simulink library "DLR_BSW_lib"  (Simulink 8.1)
settings: Solver=ode45  SolverMode=SingleTasking  StartTime=0.0  StopTime=10.0  RelTol=1e-3
settings Model: Creator=Nathan  LastModifiedBy=Nathan

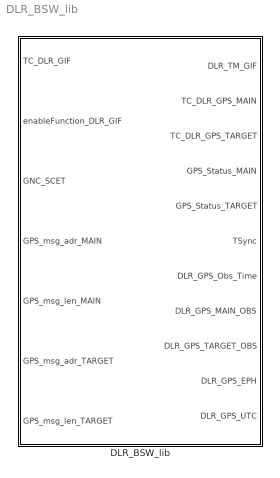
== system DLR_BSW_lib ==
  DLR_BSW_lib : Subsystem  TreatAsAtomicUnit=on  SystemSampleTime=1.0  RTWFcnName=dlr_bsw_rtw
      settings: AttributesFormatString=Priority=%<Priority>  RTWSystemCode=Nonreusable function  RTWFcnNameOpts=User specified  RTWFileNameOpts=Use function name

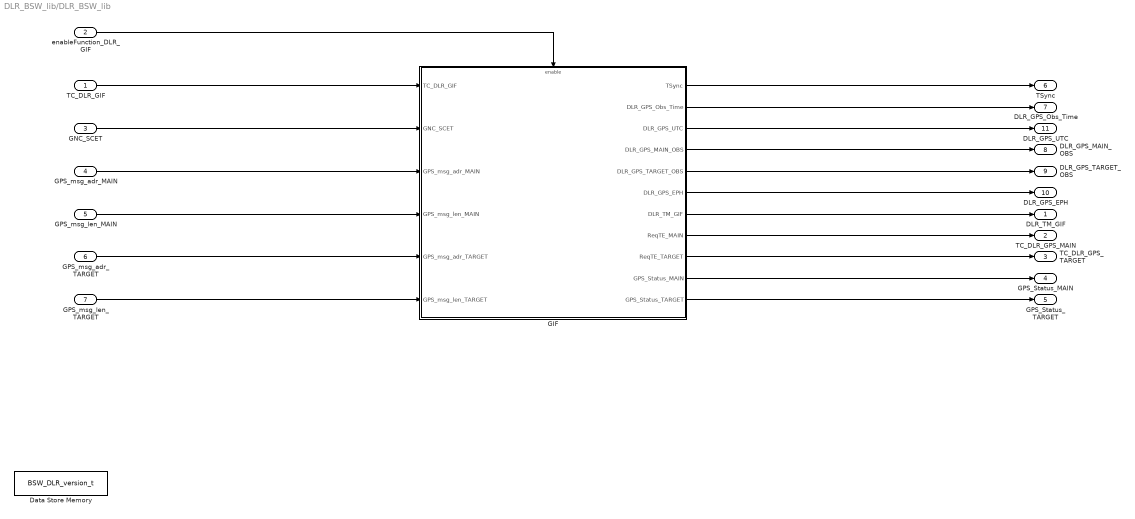
== system DLR_BSW_lib/DLR_BSW_lib ==
  TC_DLR_GIF : Inport  OutDataTypeStr=double  PortDimensions=8
  enableFunction_DLR_GIF : Inport  Port=2  OutDataTypeStr=boolean  PortDimensions=1
  GNC_SCET : Inport  Port=3  OutDataTypeStr=uint32  PortDimensions=2
  GPS_msg_adr_MAIN : Inport  Port=4  OutDataTypeStr=uint32  PortDimensions=1
  GPS_msg_len_MAIN : Inport  Port=5  OutDataTypeStr=uint32  PortDimensions=1
  GPS_msg_adr_TARGET : Inport  Port=6  OutDataTypeStr=uint32  PortDimensions=1
  GPS_msg_len_TARGET : Inport  Port=7  OutDataTypeStr=uint32  PortDimensions=1
  Data Store Memory : DataStoreMemory  DataStoreName=BSW_DLR_version_t  InitialValue=BSW_DLR_version_t  OutDataTypeStr=uint8
  GIF : Subsystem  TreatAsAtomicUnit=on
  DLR_TM_GIF : Outport  OutDataTypeStr=uint8  PortDimensions=5
  TC_DLR_GPS_MAIN : Outport  Port=2  OutDataTypeStr=uint8  PortDimensions=8
  TC_DLR_GPS_TARGET : Outport  Port=3  OutDataTypeStr=uint8  PortDimensions=8
  GPS_Status_MAIN : Outport  Port=4  OutDataTypeStr=uint8  PortDimensions=1
  GPS_Status_TARGET : Outport  Port=5  OutDataTypeStr=uint8  PortDimensions=1
  TSync : Outport  Port=6  OutDataTypeStr=uint32  PortDimensions=2
  DLR_GPS_Obs_Time : Outport  Port=7  OutDataTypeStr=uint32  PortDimensions=2
  DLR_GPS_MAIN_OBS : Outport  Port=8  OutDataTypeStr=double  PortDimensions=69
  DLR_GPS_TARGET_OBS : Outport  Port=9  OutDataTypeStr=double  PortDimensions=69
  DLR_GPS_EPH : Outport  Port=10  OutDataTypeStr=double  PortDimensions=992
  DLR_GPS_UTC : Outport  Port=11  OutDataTypeStr=uint8  PortDimensions=1
  wires:
  TC_DLR_GIF/1 -> GIF/1(TC_DLR_GIF)
  enableFunction_DLR_GIF/1 -> GIF/Enable
  GPS_msg_adr_MAIN/1 -> GIF/3(GPS_msg_adr_MAIN)
  GPS_msg_len_MAIN/1 -> GIF/4(GPS_msg_len_MAIN)
  GPS_msg_adr_TARGET/1 -> GIF/5(GPS_msg_adr_TARGET)
  GPS_msg_len_TARGET/1 -> GIF/6(GPS_msg_len_TARGET)
  GNC_SCET/1 -> GIF/2(GNC_SCET)
  GIF/7(DLR_TM_GIF) -> DLR_TM_GIF/1
  GIF/8(ReqTE_MAIN) -> TC_DLR_GPS_MAIN/1
  GIF/9(ReqTE_TARGET) -> TC_DLR_GPS_TARGET/1
  GIF/10(GPS_Status_MAIN) -> GPS_Status_MAIN/1
  GIF/11(GPS_Status_TARGET) -> GPS_Status_TARGET/1
  GIF/1(TSync) -> TSync/1
  GIF/2(DLR_GPS_Obs_Time) -> DLR_GPS_Obs_Time/1
  GIF/3(DLR_GPS_UTC) -> DLR_GPS_UTC/1
  GIF/4(DLR_GPS_MAIN_OBS) -> DLR_GPS_MAIN_OBS/1
  GIF/5(DLR_GPS_TARGET_OBS) -> DLR_GPS_TARGET_OBS/1
  GIF/6(DLR_GPS_EPH) -> DLR_GPS_EPH/1

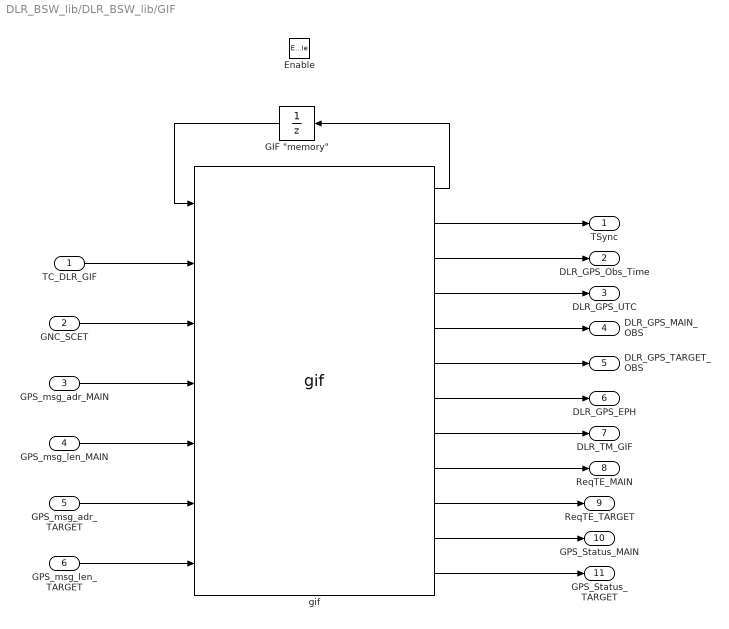
== system DLR_BSW_lib/DLR_BSW_lib/GIF ==
  TC_DLR_GIF : Inport
  GNC_SCET : Inport  Port=2
  GPS_msg_adr_MAIN : Inport  Port=3
  GPS_msg_len_MAIN : Inport  Port=4
  GPS_msg_adr_TARGET : Inport  Port=5
  GPS_msg_len_TARGET : Inport  Port=6
  Enable : EnablePort  StatesWhenEnabling=reset
  "GIF \"memory\"" : UnitDelay  SampleTime=-1
  gif : S-Function  FunctionName=gif  EnableBusSupport=off
      mask Display:
      | port_label('input',1,'MEM_in')
      | port_label('input',2,'TC_DLR_GIF')
      | port_label('input',3,'GPS_TIME')
      | port_label('input',4,'GPS_msg_adr_MAIN')
      | port_label('input',5,'GPS_msg_len_MAIN')
      | port_label('input',6,'GPS_msg_adr_TARGET')
      | port_label('input',7,'GPS_msg_len_TARGET')
      | port_label('output',1,'MEM_out')
      | port_label('output',2,'TSync')
      | port_label('output',3,'DLR_GPS_Obs_Time')
      | port_label('output',4,'DLR_GPS_UTC')
      | port_label('output',5,'DLR_GPS_MAIN_OBS')
      | port_label('output',6,'DLR_GPS_TARGET_OBS')
      | port_label('output',7,'DLR_GPS_EPH')
      | port_label('output',8,'DLR_TM_GIF')
      | port_label('output',9,'ReqTE_MAIN')
      | port_label('output',10,'ReqTE_TARGET')
      | port_label('output',11,'GPS_Status_MAIN')
      | port_label('output',12,'GPS_Status_TARGET')
  TSync : Outport  OutputWhenDisabled=reset  InitialOutput=0
  DLR_GPS_Obs_Time : Outport  Port=2  OutputWhenDisabled=reset  InitialOutput=0
  DLR_GPS_UTC : Outport  Port=3  OutputWhenDisabled=reset  InitialOutput=0
  DLR_GPS_MAIN_OBS : Outport  Port=4  OutputWhenDisabled=reset  InitialOutput=0
  DLR_GPS_TARGET_OBS : Outport  Port=5  OutputWhenDisabled=reset  InitialOutput=0
  DLR_GPS_EPH : Outport  Port=6  OutputWhenDisabled=reset  InitialOutput=0
  DLR_TM_GIF : Outport  Port=7  OutputWhenDisabled=reset  InitialOutput=0
  ReqTE_MAIN : Outport  Port=8  OutputWhenDisabled=reset  InitialOutput=0
  ReqTE_TARGET : Outport  Port=9  OutputWhenDisabled=reset  InitialOutput=0
  GPS_Status_MAIN : Outport  Port=10  OutputWhenDisabled=reset  InitialOutput=0
  GPS_Status_TARGET : Outport  Port=11  OutputWhenDisabled=reset  InitialOutput=0
  wires:
  GPS_msg_len_TARGET/1 -> gif/7
  GPS_msg_adr_TARGET/1 -> gif/6
  gif/2 -> TSync/1
  gif/3 -> DLR_GPS_Obs_Time/1
  gif/4 -> DLR_GPS_UTC/1
  gif/5 -> DLR_GPS_MAIN_OBS/1
  gif/6 -> DLR_GPS_TARGET_OBS/1
  gif/7 -> DLR_GPS_EPH/1
  gif/8 -> DLR_TM_GIF/1
  gif/9 -> ReqTE_MAIN/1
  gif/10 -> ReqTE_TARGET/1
  gif/11 -> GPS_Status_MAIN/1
  gif/12 -> GPS_Status_TARGET/1
  GPS_msg_len_MAIN/1 -> gif/5
  GPS_msg_adr_MAIN/1 -> gif/4
  GNC_SCET/1 -> gif/3
  TC_DLR_GIF/1 -> gif/2
  "GIF \"memory\""/1 -> gif/1
  gif/1 -> "GIF \"memory\""/1
